simulink model "hospital_scenario_optimisation"  (R2024b)
settings: Solver=VariableStepAuto  StartTime=0.0  StopTime=time  RelTol=1e-3
values from neighbouring files (symbols this model uses):
  m = length(data_p_arrive)    [emergency.m]
undefined symbols (not defined in the file or in its folder): entity, entitySys, get_daparture, n
settings Model: Creator=zahra  LastModifiedBy=zahra

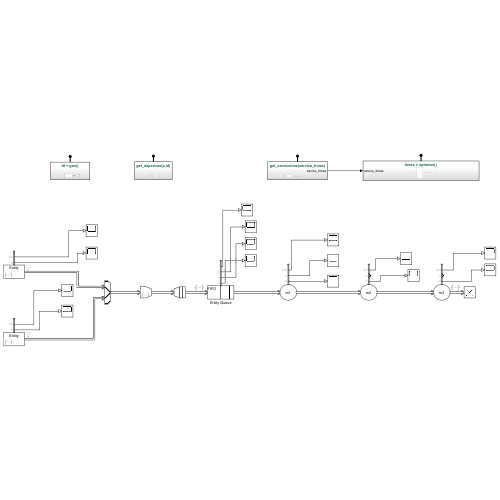
[thumbnail: Simulink's stored preview of the top-level diagram]
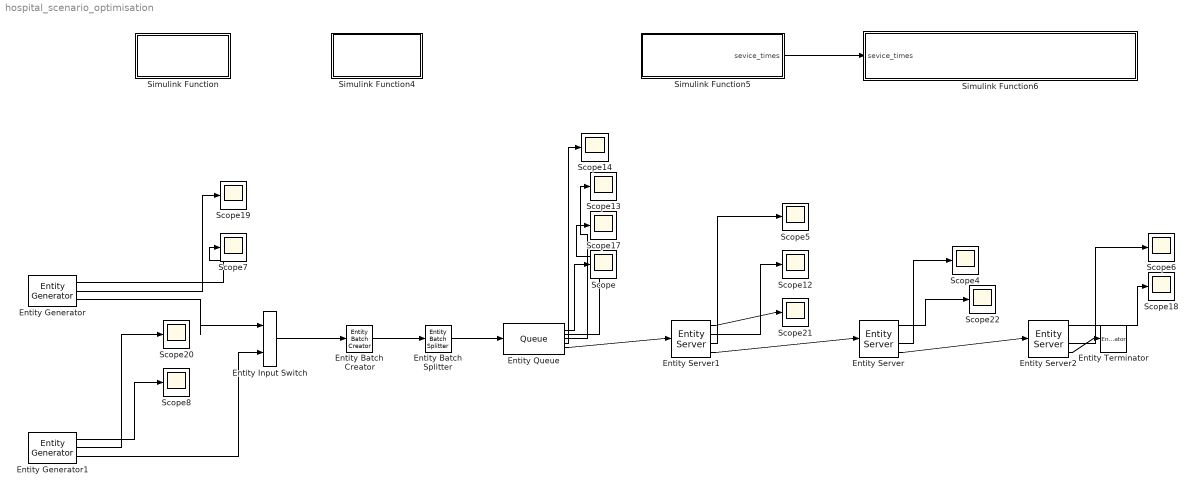
== system hospital_scenario_optimisation ==
  Entity Input Switch : EntityInputSwitch  InputPortMessageModes=m,m  OutputPortMessageModes=m
  Entity Batch Creator : EntityBatchCreator  InputPortMessageModes=m  OutputPortMessageModes=m  NumberOfEntitiesInBatch=20  BatchGenerateAction=|
      | service_times = [entity.batch.stage1; entity.batch.stage2; entity.batch.stage3]
      | get_servicetime(service_times)
      settings: OutputPortMap=o4
  Entity Batch Splitter : EntityBatchSplitter  InputPortMessageModes=m  OutputPortMessageModes=m
      settings: OutputPortMap=o4
  Entity Generator : EntityGenerator  OutputPortMessageModes=n,n,m  TimeSource=MATLAB action  IntergenerationTimeAction=dt=gen();  GenerateAction=|  AttributeName=stage1|stage2|stage3|type  AttributeInitialValue=1|2|0.5|1  NumberEntitiesDeparted=on  PendingEntityInBlock=on  EntityType=Structured  EntityTypeName=Entity
      | entity.stage1=exprnd(entity.stage1);
      | entity.stage2=exprnd(entity.stage2);
      | entity.stage3=exprnd(entity.stage3);
      settings: OutputPortMap=o0,o1,o3
  Entity Generator1 : EntityGenerator  OutputPortMessageModes=n,n,m  TimeSource=MATLAB action  IntergenerationTimeAction=dt=gen();  GenerateAction=|  AttributeName=stage1|stage2|stage3|type  AttributeInitialValue=0.5|2|1.5|2  NumberEntitiesDeparted=on  PendingEntityInBlock=on  EntityType=Structured  EntityTypeName=Entity
      | entity.stage1=exprnd(entity.stage1);
      | entity.stage2=exprnd(entity.stage2);
      | entity.stage3=exprnd(entity.stage3);
      settings: OutputPortMap=o0,o1,o3
  Entity Queue : Queue  InputPortMessageModes=m  OutputPortMessageModes=n,n,n,n,m  Capacity=Inf  EntryAction=|  NumberEntitiesDeparted=on  NumberEntitiesInBlock=on  AverageWait=on  AverageQueueLength=on
      | % Define persistent variables
      | persistent i optimiseMatrix
      | 
      | % Initialize persistent variables
      | if isempty(i)
      |     i = 0; % Initialize the persistent counter
      | end
      | 
      | if isempty(optimiseMatrix)
      |     % Initialize a fixed-size 3x20 matrix for `optimiseMatrix`
      |     % Replace the zeros with your predefined values, if available
      |     optimiseMatrix = optimise(); % [Row 1: stage1, Row 2: stage2, Row 3: stage3]
      | end
      | 
      | % Increment the persistent counter
      | i = i + 1;
      | 
      | % Ensure the index `i` does not exceed the number of columns in `optimiseMatrix`
      | if i <= size(optimiseMatrix, 2)
      |     % Assign values to entity stages using the fixed-size matrix
      |     
      |     entity.stage1 = optimiseMatrix(1, i); % Row 1, column i
      |     entity.stage2 = optimiseMatrix(2, i); % Row 2, column i
      |     entity.stage3 = optimiseMatrix(3, i); % Row 3, column i
      |     
      | else
      |     % Reset or handle end-of-loop behavior
      |     i = 0; % Reset counter if required
      | end
      settings: OutputPortMap=o0,o1,o2,o3,o5
  Entity Server : EntityServer  InputPortMessageModes=m  OutputPortMessageModes=n,n,n,m  Capacity=m2  ServiceTimeSource=Attribute  ServiceTimeAttributeName=stage2  NumberEntitiesDeparted=on  NumberEntitiesInBlock=on  Utilization=on
      settings: OutputPortMap=o0,o1,o5,o9
  Entity Server1 : EntityServer  InputPortMessageModes=m  OutputPortMessageModes=n,n,n,m  Capacity=m1  ServiceTimeSource=Attribute  ServiceTimeAttributeName=stage1  ServiceTimeAction=|  NumberEntitiesDeparted=on  NumberEntitiesInBlock=on  Utilization=on
      | % Define persistent variables
      | persistent i;
      |     
      | % Initialize the persistent variable if it's empty
      | if isempty(i)
      |    i = 1; % Start at the first index
      | end
      | 
      |  % Get stages and completion status
      | [stages, complete] = process_stage();
      | 
      | if complete==1    
      |     % Process stages if complete is 1
      |     for k = i:20
      |          dt = stages(k, 1) % Access stage data
      |                     
      |          % Increment the persistent index
      |          i = i + 1;
      |     
      |          % Exit the loop if all stages are processed
      |          if i > 20
      |               break;
      |          end
      |     end
      | end
      | dt=entity.stage1
      settings: OutputPortMap=o0,o1,o5,o9
  Entity Server2 : EntityServer  InputPortMessageModes=m  OutputPortMessageModes=n,n,n,m  Capacity=m3  ServiceTimeSource=Attribute  ServiceTimeAttributeName=stage3  ExitAction=get_daparture(entitySys.id, entity.type);  NumberEntitiesDeparted=on  NumberEntitiesInBlock=on  Utilization=on
      settings: OutputPortMap=o0,o1,o5,o9
  Entity Terminator : EntityTerminator  InputPortMessageModes=m
  Scope{,4..8,12..14,17..22} (15 alike) : Scope
  Simulink Function : Subsystem  TreatAsAtomicUnit=on
  Simulink Function4 : Subsystem  TreatAsAtomicUnit=on
  Simulink Function5 : Subsystem  TreatAsAtomicUnit=on
  Simulink Function6 : Subsystem  TreatAsAtomicUnit=on
  wires:
  Entity Generator1/3 -> Entity Input Switch/2
  Entity Server2/4 -> Entity Terminator/1
  Entity Server/3 -> Scope4/1
  Entity Server1/3 -> Scope5/1
  Entity Server2/3 -> Scope6/1
  Entity Queue/1 -> Scope/1
  Entity Generator/1 -> Scope7/1
  Entity Generator1/1 -> Scope8/1
  Entity Queue/5 -> Entity Server1/1
  Entity Server1/4 -> Entity Server/1
  Entity Server/4 -> Entity Server2/1
  Entity Server1/2 -> Scope12/1
  Entity Queue/3 -> Scope13/1
  Entity Queue/4 -> Scope14/1
  Entity Queue/2 -> Scope17/1
  Entity Generator/3 -> Entity Input Switch/1
  Entity Server2/1 -> Scope18/1
  Entity Generator/2 -> Scope19/1
  Entity Generator1/2 -> Scope20/1
  Entity Server1/1 -> Scope21/1
  Entity Server/1 -> Scope22/1
  Entity Batch Creator/1 -> Entity Batch Splitter/1
  Entity Input Switch/1 -> Entity Batch Creator/1
  Entity Batch Splitter/1 -> Entity Queue/1
  Simulink Function5/1(sevice_times) -> Simulink Function6/1(sevice_times)

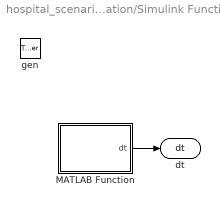
== system hospital_scenario_optimisation/Simulink Function ==
  gen : TriggerPort  TriggerType=function-call  IsSimulinkFunction=on  FunctionName=gen  FunctionVisibility=scoped  VariantControl=(inherit)
  MATLAB Function : MATLAB Function  TreatAsAtomicUnit=on
  dt : ArgOut  DisableCoverage=on  ArgumentName=dt
  wires:
  MATLAB Function/1(dt) -> dt/1

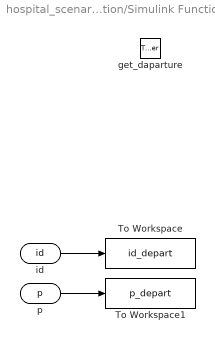
== system hospital_scenario_optimisation/Simulink Function4 ==
  get_daparture : TriggerPort  TriggerType=function-call  IsSimulinkFunction=on  FunctionName=get_daparture  FunctionVisibility=scoped  VariantControl=(inherit)
  To Workspace : ToWorkspace  VariableName=id_depart  SaveFormat=Timeseries  SampleTime=-1
  To Workspace1 : ToWorkspace  VariableName=p_depart  SaveFormat=Timeseries  SampleTime=-1
  p : ArgIn  DisableCoverage=on  ArgumentName=p
  id : ArgIn  DisableCoverage=on  Port=2  ArgumentName=id
  wires:
  p/1 -> To Workspace1/1
  id/1 -> To Workspace/1

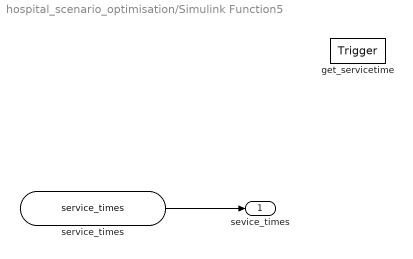
== system hospital_scenario_optimisation/Simulink Function5 ==
  get_servicetime : TriggerPort  TriggerType=function-call  IsSimulinkFunction=on  FunctionName=get_servicetime  FunctionVisibility=scoped  VariantControl=(inherit)
  service_times : ArgIn  DisableCoverage=on  PortDimensions=[3 20]  ArgumentName=service_times
  sevice_times : Outport
  wires:
  service_times/1 -> sevice_times/1

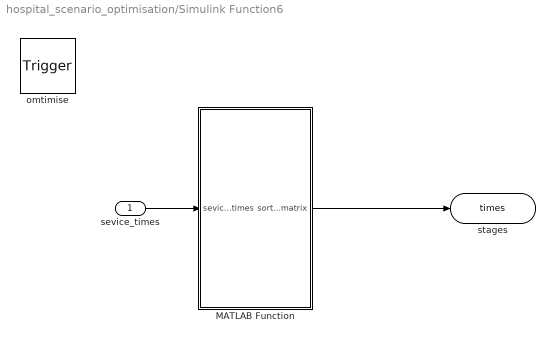
== system hospital_scenario_optimisation/Simulink Function6 ==
  sevice_times : Inport
  omtimise : TriggerPort  TriggerType=function-call  IsSimulinkFunction=on  FunctionName=optimise  FunctionVisibility=scoped  VariantControl=(inherit)
  MATLAB Function : MATLAB Function  TreatAsAtomicUnit=on
  stages : ArgOut  DisableCoverage=on  PortDimensions=[3,20]  ArgumentName=times
  wires:
  sevice_times/1 -> MATLAB Function/1(sevice_times)
  MATLAB Function/1(sorted_matrix) -> stages/1

== matlab function hospital_scenario_optimisation/Simulink Function/MATLAB Function ==
  data: dt output
function dt = fcn()

persistent count; % Declare a persistent variable to track entities
if isempty(count)
    count = 0; % Initialize count at the start of the simulation
end
if count < 18
    dt = 0; % Generate entities with no delay
    count = count + 1; % Increment the count
else
    dt = Inf; % Stop further entity generation
end

== matlab function hospital_scenario_optimisation/Simulink Function6/MATLAB Function ==
  data: sorted_matrix output; sevice_times input
function sorted_matrix = fcn(sevice_times)

    column_sums = sum(sevice_times, 1);
    
    % Sort the column sums and get the sorting indices
    [~, sort_indices] = sort(column_sums, 'ascend');
    
    % Rearrange the matrix columns based on the sorting indices
    sorted_matrix = sevice_times(:, sort_indices)
end
